simulink model "dev_AirSide"  (R2020b)
settings: Solver=VariableStepAuto  StartTime=0.0  StopTime=800  RelTol=1e-3
model workspace (MAT data in the model file):
  G_sup_tsp = Simulink.Signal
  G_sup_tsp.DataType = 'double'
  G_sup_tsp.Dimensions = -1
  G_sup_tsp.DimensionsMode = 'auto'
  G_sup_tsp.Complexity = 'real'
  G_sup_tsp.SampleTime = -1
  G_sup_tsp.SamplingMode = 'auto'
  G_sup_tsp.InitialValue = '175'
libraries: simulink_extras x1
settings Model: Creator=Mr_Li  LastModifiedBy=Mr_Li

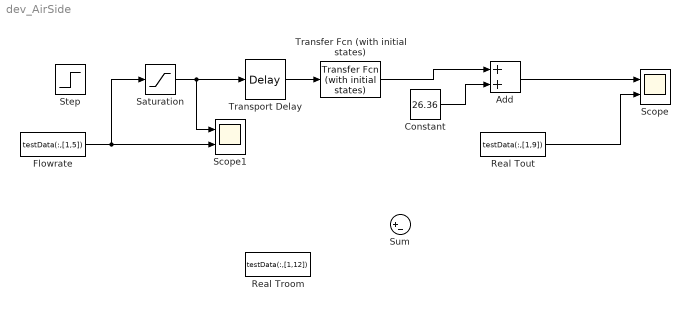
== system dev_AirSide ==
  Add : Sum
  Constant : Constant  Value=26.36
  Flowrate : FromWorkspace  VariableName=testData(:,[1,5])  SampleTime=1
  Real Tout : FromWorkspace  VariableName=testData(:,[1,9])
  Real Troom : FromWorkspace  VariableName=testData(:,[1,12])
  Saturation : Saturate  UpperLimit=0.75  LowerLimit=0
  Scope : Scope  NumInputPorts=2
  Scope1 : Scope  NumInputPorts=2
  Step : Step  Time=35  After=0.75  SampleTime=0
  Sum : Sum  Inputs=|+-
  Transfer Fcn (with initial states) : simulink_extras/Additional Linear/Transfer Fcn (with initial states)  N=[60]  D="[27  1]"  X0=0
  Transport Delay : TransportDelay
  wires:
  Real Tout/1 -> Scope/2
  Add/1 -> Scope/1
  Transfer Fcn (with initial states)/1 -> Add/1
  Constant/1 -> Add/2
  Flowrate/1 -> Scope1/2, Saturation/1
  Saturation/1 -> Transport Delay/1, Scope1/1
  Transport Delay/1 -> Transfer Fcn (with initial states)/1
